simulink model "lookup_nD_TestGen36"  (R2017b)
settings: Solver=FixedStepDiscrete  StartTime=0.0  StopTime=10.0  RelTol=1e-3
model workspace (MAT data in the model file):
  LUTObjLKnD36 = Simulink.LookupTable
  LUTObjLKnD36.Table = Simulink.lookuptable.Table
  LUTObjLKnD36.Table.Value = reshape([4 16 10 4 16 10 4 16 10 4 16 10 4 16 10 4 16 10 5 19 18 5 19 18 5 19 18 5 19 18 5 19 18 5 19 18 6 20 23 6 20 23 6 20 23 6 20 23 6 20 23 6 20 23 7 21 24 7 21 24 7 21 24 7 21 24 7 21 24 7 21 24 8 22 25 8 22 25 8 22 25 8 22 25 8 22 25 8 22 25 4 16 10 4 16 10 4 16 10 4 16 10 4 16 10 4 16 10 5 19 18 5 19 18 5 19 18 5 19 18 5 19 18 5 19 18 6 20 23 6 20 23 6 20 23 6 20 23 6 20 23 6 20 23 7 21 24 7 21 24 7 21 24 7 21 24 7 21 24 7 21 24 8 22 25 8 22 25 8 22 25 8 22 25 8 22 25 8 22 25 4 16 10 4 16 10 4 16 10 4 16 10 4 16 10 4 16 10 5 19 18 5 19 18 5 19 18 5 19 18 5 19 18 5 19 18 6 20 23 6 20 23 6 20 23 6 20 23 6 20 23 6 20 23 7 21 24 7 21 24 7 21 24 7 21 24 7 21 24 7 21 24 8 22 25 8 22 25 8 22 25 8 22 25 8 22 25 8 22 25 4 16 10 4 16 10 4 16 10 4 16 10 4 16 10 4 16 10 5 19 18 5 19 18 5 19 18 5 19 18 5 19 18 5 19 18 6 20 23 6 20 23 6 20 23 6 20 23 6 20 23 6 20 23 7 21 24 7 21 24 7 21 24 7 21 24 7 21 24 7 21 24 8 22 25 8 22 25 8 22 25 8 22 25 8 22 25 8 22 25 4 16 10 4 16 10 4 16 10 4 16 10 4 16 10 4 16 10 5 19 18 5 19 18 5 19 18 5 19 18 5 19 18 5 19 18 6 20 23 6 20 23 6 20 23 6 20 23 6 20 23 6 20 23 7 21 24 7 21 24 7 21 24 7 21 24 7 21 24 7 21 24 8 22 25 8 22 25 8 22 25 8 22 25 8 22 25 8 22 25 4 16 10 4 16 10 4 16 10 4 16 10 4 16 10 4 16 10 5 19 18 5 19 18 5 19 18 5 19 18 5 19 18 5 19 18 6 20 23 6 20 23 6 20 23 6 20 23 6 20 23 6 20 23 7 21 24 7 21 24 7 21 24 7 21 24 7 21 24 7 21 24 8 22 25 8 22 25 8 22 25 8 22 25 8 22 25 8 22 25 4 16 10 4 16 10 4 16 10 4 16 10 4 16 10 4 16 10 5 19 18 5 19 18 5 19 18 5 19 18 5 19 18 5 19 18 6 20 23 6 20 23 6 20 23 6 20 23 6 20 23 6 20 23 7 21 24 7 21 24 7 21 24 7 21 24 7 21 24 7 21 24 8 22 25 8 22 25 8 22 25 8 22 25 8 22 25 8 22 25 4 16 10 4 16 10 4 16 10 4 16 10 4 16 10 4 16 10 5 19 18 5 19 18 5 19 18 5 19 18 5 19 18 5 19 18 6 20 23 6 20 23 6 20 23 6 20 23 6 20 23 6 20 23 7 21 24 7 21 24 7 21 24 7 21 24 7 21 24 7 21 24 8 22 25 8 22 25 8 22 25 8 22 25 8 22 25 8 22 25], [2 5 3 2 3 4])
  LUTObjLKnD36.Table.Dimensions = [2 5 3 2 3 4]
  LUTObjLKnD36.Table.DataType = 'auto'
  LUTObjLKnD36.Table.FieldName = 'Table'
  LUTObjLKnD36.BreakpointsSpecification = 'Even spacing'
  LUTObjLKnD36.Breakpoints(1) = Simulink.lookuptable.Evenspacing
  LUTObjLKnD36.Breakpoints(1).FirstPoint = 109.293918974
  LUTObjLKnD36.Breakpoints(1).Spacing = 1.5
  LUTObjLKnD36.Breakpoints(1).FirstPointName = 'BPFirstPoint1'
  LUTObjLKnD36.Breakpoints(1).SpacingName = 'BPSpacing1'
  LUTObjLKnD36.Breakpoints(1).TunableSizeName = 'N1'
  LUTObjLKnD36.Breakpoints(1).DataType = 'auto'
  LUTObjLKnD36.Breakpoints(1).FieldName = 'BP1'
  LUTObjLKnD36.Breakpoints(2) = Simulink.lookuptable.Evenspacing
  LUTObjLKnD36.Breakpoints(2).FirstPoint = 16.3049102694
  LUTObjLKnD36.Breakpoints(2).Spacing = 1.5
  LUTObjLKnD36.Breakpoints(2).FirstPointName = 'BPFirstPoint2'
  LUTObjLKnD36.Breakpoints(2).SpacingName = 'BPSpacing2'
  LUTObjLKnD36.Breakpoints(2).TunableSizeName = 'N2'
  LUTObjLKnD36.Breakpoints(2).DataType = 'auto'
  LUTObjLKnD36.Breakpoints(2).FieldName = 'BP2'
  LUTObjLKnD36.Breakpoints(3) = Simulink.lookuptable.Evenspacing
  LUTObjLKnD36.Breakpoints(3).FirstPoint = 103.834522697
  LUTObjLKnD36.Breakpoints(3).Spacing = 1.5
  LUTObjLKnD36.Breakpoints(3).FirstPointName = 'BPFirstPoint3'
  LUTObjLKnD36.Breakpoints(3).SpacingName = 'BPSpacing3'
  LUTObjLKnD36.Breakpoints(3).TunableSizeName = 'N3'
  LUTObjLKnD36.Breakpoints(3).DataType = 'auto'
  LUTObjLKnD36.Breakpoints(3).FieldName = 'BP3'
  LUTObjLKnD36.Breakpoints(4) = Simulink.lookuptable.Evenspacing
  LUTObjLKnD36.Breakpoints(4).FirstPoint = 109.166395804
  LUTObjLKnD36.Breakpoints(4).Spacing = 1.5
  LUTObjLKnD36.Breakpoints(4).FirstPointName = 'BPFirstPoint4'
  LUTObjLKnD36.Breakpoints(4).SpacingName = 'BPSpacing4'
  LUTObjLKnD36.Breakpoints(4).TunableSizeName = 'N4'
  LUTObjLKnD36.Breakpoints(4).DataType = 'auto'
  LUTObjLKnD36.Breakpoints(4).FieldName = 'BP4'
  LUTObjLKnD36.Breakpoints(5) = Simulink.lookuptable.Evenspacing
  LUTObjLKnD36.Breakpoints(5).FirstPoint = 63.16905054
  LUTObjLKnD36.Breakpoints(5).Spacing = 1.5
  LUTObjLKnD36.Breakpoints(5).FirstPointName = 'BPFirstPoint5'
  LUTObjLKnD36.Breakpoints(5).SpacingName = 'BPSpacing5'
  LUTObjLKnD36.Breakpoints(5).TunableSizeName = 'N5'
  LUTObjLKnD36.Breakpoints(5).DataType = 'auto'
  LUTObjLKnD36.Breakpoints(5).FieldName = 'BP5'
  LUTObjLKnD36.Breakpoints(6) = Simulink.lookuptable.Evenspacing
  LUTObjLKnD36.Breakpoints(6).FirstPoint = 110.795811235
  LUTObjLKnD36.Breakpoints(6).Spacing = 1.5
  LUTObjLKnD36.Breakpoints(6).FirstPointName = 'BPFirstPoint6'
  LUTObjLKnD36.Breakpoints(6).SpacingName = 'BPSpacing6'
  LUTObjLKnD36.Breakpoints(6).TunableSizeName = 'N6'
  LUTObjLKnD36.Breakpoints(6).DataType = 'auto'
  LUTObjLKnD36.Breakpoints(6).FieldName = 'BP6'
  LUTObjLKnD36.SupportTunableSize = 0
  LUTObjLKnD36.StructTypeInfo = Simulink.lookuptable.StructTypeInfo
  LUTObjLKnD36.StructTypeInfo.Name = 'LUT'
  LUTObjLKnD36.StructTypeInfo.DataScope = 'Auto'
settings Model: Creator=ktrinh  LastModifiedBy=ktrinh
settings DebuggingCC: ParameterOverflowMsg=none

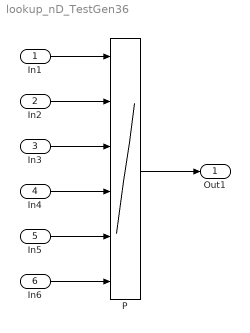
== system lookup_nD_TestGen36 ==
  In1 : Inport  OutMin=0  OutMax=127  PortDimensions=1
  In2 : Inport  Port=2  OutMin=0  OutMax=127
  In3 : Inport  Port=3  OutMin=0  OutMax=127
  In4 : Inport  Port=4  OutMin=0  OutMax=127
  In5 : Inport  Port=5  OutMin=0  OutMax=127
  In6 : Inport  Port=6  OutMin=0  OutMax=127
  P : Lookup_n-D  NumberOfTableDimensions=6  DataSpecification=Lookup table object  LookupTableObject=LUTObjLKnD36  BreakpointsSpecification=Even spacing  BreakpointsForDimension3=[5, 7]  Table=reshape(repmat([4 5 6;16 19 20;10 18 23],1,2),[3,3,2])  UseLastTableValue=on  InternalRulePriority=Speed  RndMeth=Simplest  InputSameDT=on
  Out1 : Outport
  wires:
  In1/1 -> P/1
  In2/1 -> P/2
  In3/1 -> P/3
  In4/1 -> P/4
  In5/1 -> P/5
  In6/1 -> P/6
  P/1 -> Out1/1
